simulink model "observer_img"  (R2012b)
settings: Solver=ode45  StartTime=0.0  StopTime=10.0  RelTol=1e-3
undefined symbols (not defined in the file or in its folder): A_obs, B_obs, C_obs, K_c, l
settings Model: Creator=rasme879  LastModifiedBy=rasme879

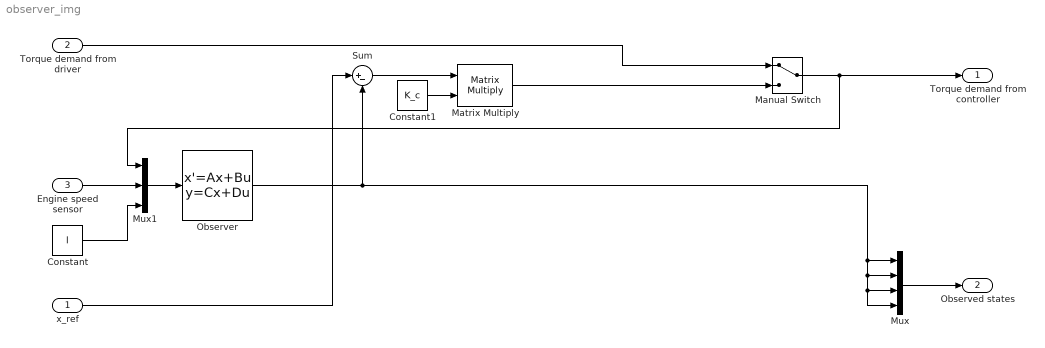
== system observer_img ==
  x_ref : Inport
  Torque demand from driver : Inport  Port=2
  Engine speed sensor : Inport  Port=3
  Constant : Constant  Value=l
  Constant1 : Constant  Value=K_c
  Manual Switch : ManualSwitch
  Matrix Multiply : Product  Multiplication=Matrix(*)
  Mux : Mux
  Mux1 : Mux  Inputs=3
  Observer : StateSpace  A=A_obs  B=B_obs  C=C_obs  D=zeros(size(B_obs))
  Sum : Sum  Inputs=|+-
  Torque demand from controller : Outport
  Observed states : Outport  Port=2
  wires:
  Manual Switch/1 -> Mux1/1, Torque demand from controller/1
  Engine speed sensor/1 -> Mux1/2
  x_ref/1 -> Sum/1
  Matrix Multiply/1 -> Manual Switch/2
  Observer/1 -> Mux/3, Mux/4, Mux/2, Mux/1, Sum/2
  Mux/1 -> Observed states/1
  Mux1/1 -> Observer/1
  Constant/1 -> Mux1/3
  Sum/1 -> Matrix Multiply/1
  Torque demand from driver/1 -> Manual Switch/1
  Constant1/1 -> Matrix Multiply/2
